simulink model "testVectorSensor"  (R2019b)
settings: configuration reference "cset" (kept outside this file)
PreLoadFcn:
  | disp(['Executing PreLoadFcn in ' get_param(gcs,'Name')])
  | 
  | % Path
  | addpath(fullfile('..','mdl'));
  | 
  | % Load configuration
  | load('testvectorsensor_cset');
  | 
  | % Load bus objects
  | load('SonarWorkbenchPublicBusObjects');
StopFcn:
  | disp(['Executing StopFcn in ' get_param(gcs,'Name')])
  | 
  | % Plot beam pattern
  | PlotNEDaxes(0,0,0)
  | Plot3DBP(theta,psi,BP,[],[],gca)
model workspace (MAT data in the model file):
  Ne = 4
  Ntype = 2
settings Model: Creator=tom  LastModifiedBy=tom
settings ConfigSetRef: SourceName=cset  SourceLocation=Base Workspace

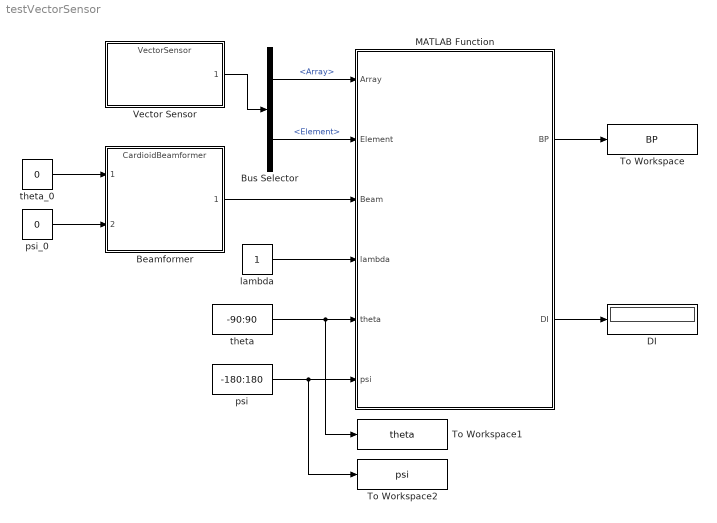
== system testVectorSensor ==
  Beamformer : ModelReference  ModelNameDialog=CardioidBeamformer  ModelReferenceVersion=1.11
      mask Display:
      | % Cover port labels
      | patch([0 1 1 0],[0.1 0.1 0.8 0.8],[0.910 0.820 0.322])
      | 
      | % Plot cardioid
      | a = 0.2;
      | th = 0:360;
      | r = a + a*cosd(th);
      | x = 0.5-a+r.*cosd(th);
      | y = 0.5+r.*sind(th);
      | patch(x,y,[0.5 0.5 1])
      | plot(x,y)
      | 
      | % Label Ports
      | port_label('input',1,'\theta_0','interpreter','tex')
      | port_label('input',2,'\psi_0','interpreter','tex')
      | port_label('output',1,'Beam','interpreter','tex')
  Bus Selector : BusSelector  OutputSignals=Array,Element
  DI : Display
  MATLAB Function : MATLAB Function  TreatAsAtomicUnit=on
  To Workspace : ToWorkspace  VariableName=BP  SampleTime=-1
      settings: MaxDataPoints=1
  To Workspace1 : ToWorkspace  VariableName=theta  SampleTime=-1
      settings: MaxDataPoints=1
  To Workspace2 : ToWorkspace  VariableName=psi  SampleTime=-1
      settings: MaxDataPoints=1
  Vector Sensor : ModelReference  ModelNameDialog=VectorSensor  ModelReferenceVersion=1.15
  lambda : Constant  OutDataTypeStr=double
  psi : Constant  Value=-180:180  OutDataTypeStr=double
  psi_0 : Constant  Value=0  OutDataTypeStr=double
  theta : Constant  Value=-90:90  OutDataTypeStr=double
  theta_0 : Constant  Value=0  OutDataTypeStr=double
  wires:
  theta_0/1 -> Beamformer/1
  psi_0/1 -> Beamformer/2
  Vector Sensor/1 -> Bus Selector/1
  Bus Selector/1 -> MATLAB Function/1(Array)  "<Array>"
  Bus Selector/2 -> MATLAB Function/2(Element)  "<Element>"
  Beamformer/1 -> MATLAB Function/3(Beam)
  lambda/1 -> MATLAB Function/4(lambda)
  theta/1 -> To Workspace1/1, MATLAB Function/5(theta)
  psi/1 -> To Workspace2/1, MATLAB Function/6(psi)
  MATLAB Function/1(BP) -> To Workspace/1
  MATLAB Function/2(DI) -> DI/1

== matlab function testVectorSensor/MATLAB Function ==
  data: Array input Bus: SonarWorkbenchArrayObj; BP output double size=[181 361]; Element input Bus: SonarWorkbenchElementObj; Beam input Bus: SonarWorkbenchBeamObj; lambda input double size=1; theta input double size=181; psi input double size=361; DI output
function [BP,DI] = EvaluateBeamPattern(Array,Element,Beam,lambda,theta,psi)
%#codegen
Ntheta = length(theta);
Npsi = length(psi);
tmp = BeamPattern(Array,Element,Beam,lambda,theta,psi);
BP = tmp(1:Ntheta,1:Npsi);
DI = CalculateDI(theta,psi,BP);
